simulink model "lin_controlsys_altitude"  (R2019b)
settings: Solver=VariableStepAuto  StartTime=0.0  StopTime=10.0  RelTol=1e-3
values from neighbouring files (symbols this model uses):
  A2 = [0  0; 1  0]    [ss_model_altitude.mat]
  B2 = [1 0]    [ss_model_altitude.mat]
  Ts = 0.001    [main_rocketmodel.m]    (also in main_sim_rocket.m; sim_lin.m; square_sig.m; sum_squares_sig.m)
undefined symbols (not defined in the file or in its folder): K2
settings Model: Creator=bia  LastModifiedBy=bia
settings DataIOCC: ExternalInput=[t_signal, x_3]  LoadExternalInput=on

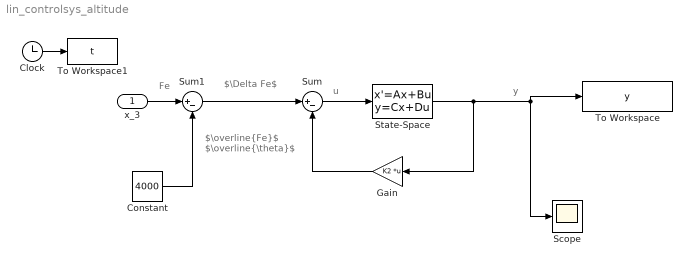
== system lin_controlsys_altitude ==
  note: $\Delta Fe$
  note: y
  note: u
  note: $\overline{Fe}$ $\overline{\theta}$
  note: Fe
  x_3 : Inport
  Clock : Clock
  Constant : Constant  Value=4000  SampleTime=Ts
  Gain : Gain  Gain=K2  Multiplication=Matrix(K*u)
  Scope : Scope
  State-Space : StateSpace  A=A2  B=B2  C=eye(2)  D=[0; 0]  InitialCondition=0
  Sum : Sum  Inputs=|+-
  Sum1 : Sum  Inputs=|+-
  To Workspace : ToWorkspace  VariableName=y  SampleTime=Ts
  To Workspace1 : ToWorkspace  VariableName=t  SampleTime=Ts
  wires:
  Sum/1 -> State-Space/1
  Gain/1 -> Sum/2
  State-Space/1 -> Gain/1, Scope/1, To Workspace/1
  Sum1/1 -> Sum/1
  x_3/1 -> Sum1/1
  Clock/1 -> To Workspace1/1
  Constant/1 -> Sum1/2
